simulink model "VCU_SW_1"  (R2023b)
settings: Solver=FixedStepDiscrete  StartTime=0.0  StopTime=inf  FixedStep=1e-2  RelTol=1e-3
PreLoadFcn:
  | RTWConfigurationCB('preloadfcn', bdroot);
InitFcn:
  | loadvar_ttc500
undefined symbols (not defined in the file): BrkPedalTypes, CabMovModeTypes, cFuseTempSensAcc_X, cFuseTempSensAcc_Y, cFuseTempSensVal_X, cFuseTempSensVal_Y, cTMSTempSensVal_X, cTMSTempSensVal_Y, cTransferCaseSpeedRatio, diag_state, DoorsPositionTypes, dP_filter_Y, DriverOccClassSystemTypes, ErrorValueTypes, fatal_error_callback, IO_ADC_NO_RANGE, LadderStatusTypes, pAnalogCabRotSensAcc, pAnalogCabRotSensMaxVolt, pAnalogCabRotSensMinVolt, pAnalogCabRotSensRange, pAnalogCabRotSensZeroVolt, pBrkActivePress, pCabTiltSensAcc, pCabTiltSensMaxCur, pCabTiltSensMinCur, pDistanceCorrection, pECANManual_BPNEnable, pECANManual_BPNEnabler_Flag, pFilterSensAccRes, pHDirMaxDiffFrq, pHDirSensHighLvl, pHDirSensLowLvl, pMainGearRatio, pMaxFilterSensRes, pMaxFirstPedalSensValue, pMaxFuseTempSensRes, pMaxPressLoss, pMaxPressSensCurrent, pMaxPressValue, pMaxPressValueHydMotAndPump, pMaxPressValueParkDrain, pMaxSecondPedalSensValue, pMaxTempSensVoltage, pMaxTempValue, pMaxTMSTempSensRes, pMinFilterSensRes, pMinFirstPedalSensValue, pMinFuseTempSensRes, pMinPressLoss, pMinPressSensCurrent, pMinPressValue, pMinSecondPedalSensValue, pMinTempSensVoltage, pMinTempValue, pMinTMSTempSensRes, pMotorRingTeethNum, pPedalSensAccuracyPct, pPedalSensAccuracyVolt, pPressLossTreshhold ... (+20)
libraries: TTlibrary x270, canmsglib x127, simulink x88
(part 11 of 19)

== system VCU_SW_1/logSignal/getListData/pageHighvoltageAppData/getListDataII8 ==
  getListDataII8 : TriggerPort  TriggerType=function-call  IsSimulinkFunction=on  FunctionName=getListDataII8  FunctionVisibility=scoped  VariantControl=(inherit)
  Constant : Constant  Value=uint8(6)
  Data Store Read1 : DataStoreRead  DataStoreName=sMinCellVoltage  IndexOptions=Index vector (dialog)  Indices=1  OutputSizes=1
  Data Store Read2 : DataStoreRead  DataStoreName=sMaxBatTemp  IndexOptions=Index vector (dialog)  Indices=1  OutputSizes=1
  Data Store Read3 : DataStoreRead  DataStoreName=sMinBatTemp  IndexOptions=Index vector (dialog)  Indices=1  OutputSizes=1
  Demux1 : Demux  Outputs=2
  Demux11 : Demux  Outputs=2
  Demux2 : Demux  Outputs=2
  Function Caller : FunctionCaller  FunctionPrototype=data = getListData.splitIntoTwoBytes(value)  InputArgumentSpecifications=<Enter example>  OutputArgumentSpecifications=<Enter example>
  Function Caller1 : FunctionCaller  FunctionPrototype=data = getListData.splitIntoTwoBytes(value)  InputArgumentSpecifications=<Enter example>  OutputArgumentSpecifications=<Enter example>
  Function Caller2 : FunctionCaller  FunctionPrototype=data = getListData.splitIntoTwoBytes(value)  InputArgumentSpecifications=<Enter example>  OutputArgumentSpecifications=<Enter example>
  Ground : Ground
  Mux : Mux  Inputs=7
  data : ArgOut  DisableCoverage=on  OutDataTypeStr=uint8  PortDimensions=[1,7]  ArgumentName=data
  len : ArgOut  Port=2  OutDataTypeStr=uint8  ArgumentName=len
  wires:
  Mux/1 -> data/1
  Constant/1 -> len/1
  Function Caller/1 -> Demux11/1
  Demux11/1 -> Mux/1
  Data Store Read1/1 -> Function Caller/1
  Demux11/2 -> Mux/2
  Demux1/2 -> Mux/4
  Data Store Read2/1 -> Function Caller1/1
  Demux1/1 -> Mux/3
  Function Caller1/1 -> Demux1/1
  Function Caller2/1 -> Demux2/1
  Demux2/2 -> Mux/6
  Demux2/1 -> Mux/5
  Ground/1 -> Mux/7
  Data Store Read3/1 -> Function Caller2/1

== system VCU_SW_1/logSignal/getListData/pageHighvoltageAppData/getListDataII9 ==
  getListDataII9 : TriggerPort  TriggerType=function-call  IsSimulinkFunction=on  FunctionName=getListDataII9  FunctionVisibility=scoped  VariantControl=(inherit)
  Constant : Constant  Value=uint8(6)
  Data Store Read1 : DataStoreRead  DataStoreName=sTotalVoltage  IndexOptions=Index vector (dialog)  Indices=1  OutputSizes=1
  Data Store Read2 : DataStoreRead  DataStoreName=sMaxCellVoltTemp  IndexOptions=Index vector (dialog)  Indices=1  OutputSizes=1
  Data Store Read3 : DataStoreRead  DataStoreName=sMinCellVoltTemp  IndexOptions=Index vector (dialog)  Indices=1  OutputSizes=1
  Data Store Read4 : DataStoreRead  DataStoreName=sSettingTargetWaterTemp  IndexOptions=Index vector (dialog)  Indices=1  OutputSizes=1
  Data Store Read5 : DataStoreRead  DataStoreName=sAverageBatTemp  IndexOptions=Index vector (dialog)  Indices=1  OutputSizes=1
  Demux11 : Demux  Outputs=2
  Function Caller : FunctionCaller  FunctionPrototype=data = getListData.splitIntoTwoBytes(value)  InputArgumentSpecifications=<Enter example>  OutputArgumentSpecifications=<Enter example>
  Ground : Ground
  Mux : Mux  Inputs=7
  data : ArgOut  DisableCoverage=on  OutDataTypeStr=uint8  PortDimensions=[1,7]  ArgumentName=data
  len : ArgOut  Port=2  OutDataTypeStr=uint8  ArgumentName=len
  wires:
  Data Store Read1/1 -> Function Caller/1
  Function Caller/1 -> Demux11/1
  Constant/1 -> len/1
  Mux/1 -> data/1
  Demux11/1 -> Mux/3
  Demux11/2 -> Mux/4
  Data Store Read3/1 -> Mux/2
  Data Store Read2/1 -> Mux/1
  Data Store Read4/1 -> Mux/5
  Data Store Read5/1 -> Mux/6
  Ground/1 -> Mux/7

== system VCU_SW_1/logSignal/getListData/pageOutputRawData/getListDataOI1 ==
  getListDataOI1 : TriggerPort  TriggerType=function-call  IsSimulinkFunction=on  FunctionName=getListDataOI1  FunctionVisibility=scoped  VariantControl=(inherit)
  Data Store Read2 : DataStoreRead  DataStoreName=sCoolSensSup  IndexOptions=Index vector (dialog)  Indices=1  OutputSizes=1
  Data Store Read3 : DataStoreRead  DataStoreName=sOnBrdChrgTermSttSup  IndexOptions=Index vector (dialog)  Indices=1  OutputSizes=1
  Data Store Read4 : DataStoreRead  DataStoreName=sHVILSup  IndexOptions=Index vector (dialog)  Indices=1  OutputSizes=1
  Data Store Read5 : DataStoreRead  DataStoreName=sOnBrdFastChrgSup  IndexOptions=Index vector (dialog)  Indices=1  OutputSizes=1
  Data Store Read6 : DataStoreRead  DataStoreName=sPressSensSup  IndexOptions=Index vector (dialog)  Indices=1  OutputSizes=1
  Data Store Read7 : DataStoreRead  DataStoreName=sGearboxSensSup  IndexOptions=Index vector (dialog)  Indices=1  OutputSizes=1
  Data Store Read8 : DataStoreRead  DataStoreName=sACDCChrgConvSwt  IndexOptions=Index vector (dialog)  Indices=1  OutputSizes=1
  Mux : Mux  Inputs=7
  data : ArgOut  DisableCoverage=on  OutDataTypeStr=uint8  PortDimensions=[1,7]  ArgumentName=data
  wires:
  Mux/1 -> data/1
  Data Store Read2/1 -> Mux/7
  Data Store Read3/1 -> Mux/6
  Data Store Read8/1 -> Mux/1
  Data Store Read4/1 -> Mux/5
  Data Store Read7/1 -> Mux/2
  Data Store Read5/1 -> Mux/4
  Data Store Read6/1 -> Mux/3

== system VCU_SW_1/logSignal/getListData/pageOutputRawData/getListDataOI2 ==
  getListDataOI2 : TriggerPort  TriggerType=function-call  IsSimulinkFunction=on  FunctionName=getListDataOI2  FunctionVisibility=scoped  VariantControl=(inherit)
  Data Store Read : DataStoreRead  DataStoreName=sCapsSup  IndexOptions=Index vector (dialog)  Indices=1  OutputSizes=1
  Data Store Read1 : DataStoreRead  DataStoreName=sPumpFlowSetPnt  IndexOptions=Index vector (dialog)  Indices=1  OutputSizes=1
  Data Store Read12 : DataStoreRead  DataStoreName=sTMSComprSetPnt  IndexOptions=Index vector (dialog)  Indices=1  OutputSizes=1
  Data Store Read13 : DataStoreRead  DataStoreName=sCircPumpSetPnt  IndexOptions=Index vector (dialog)  Indices=1  OutputSizes=1
  Demux : Demux  Outputs=2
  Demux1 : Demux  Outputs=2
  Demux2 : Demux  Outputs=2
  Function Caller3 : FunctionCaller  FunctionPrototype=data = getListData.splitIntoTwoBytes(value)  InputArgumentSpecifications=<Enter example>  OutputArgumentSpecifications=<Enter example>
  Function Caller4 : FunctionCaller  FunctionPrototype=data = getListData.splitIntoTwoBytes(value)  InputArgumentSpecifications=<Enter example>  OutputArgumentSpecifications=<Enter example>
  Function Caller5 : FunctionCaller  FunctionPrototype=data = getListData.splitIntoTwoBytes(value)  InputArgumentSpecifications=<Enter example>  OutputArgumentSpecifications=<Enter example>
  Mux1 : Mux  Inputs=7
  data : ArgOut  DisableCoverage=on  OutDataTypeStr=uint8  PortDimensions=[1,7]  ArgumentName=data
  wires:
  Mux1/1 -> data/1
  Data Store Read12/1 -> Function Caller4/1
  Demux1/1 -> Mux1/3
  Demux/2 -> Mux1/2
  Demux2/1 -> Mux1/5
  Demux/1 -> Mux1/1
  Data Store Read13/1 -> Function Caller5/1
  Demux2/2 -> Mux1/6
  Function Caller3/1 -> Demux/1
  Data Store Read1/1 -> Function Caller3/1
  Data Store Read/1 -> Mux1/7
  Demux1/2 -> Mux1/4
  Function Caller4/1 -> Demux1/1
  Function Caller5/1 -> Demux2/1

== system VCU_SW_1/logSignal/getListData/pageOutputRawData/getListDataOI3 ==
  getListDataOI3 : TriggerPort  TriggerType=function-call  IsSimulinkFunction=on  FunctionName=getListDataOI3  FunctionVisibility=scoped  VariantControl=(inherit)
  Data Store Read10 : DataStoreRead  DataStoreName=sSecondGearVlvSetPnt  IndexOptions=Index vector (dialog)  Indices=1  OutputSizes=1
  Data Store Read11 : DataStoreRead  DataStoreName=sRemBrkVlvSetPnt  IndexOptions=Index vector (dialog)  Indices=1  OutputSizes=1
  Data Store Read9 : DataStoreRead  DataStoreName=sFirstGearVlvSetPnt  IndexOptions=Index vector (dialog)  Indices=1  OutputSizes=1
  Demux3 : Demux  Outputs=2
  Demux4 : Demux  Outputs=2
  Demux5 : Demux  Outputs=2
  Function Caller : FunctionCaller  FunctionPrototype=data = getListData.splitIntoTwoBytes(value)  InputArgumentSpecifications=<Enter example>  OutputArgumentSpecifications=<Enter example>
  Function Caller1 : FunctionCaller  FunctionPrototype=data = getListData.splitIntoTwoBytes(value)  InputArgumentSpecifications=<Enter example>  OutputArgumentSpecifications=<Enter example>
  Function Caller2 : FunctionCaller  FunctionPrototype=data = getListData.splitIntoTwoBytes(value)  InputArgumentSpecifications=<Enter example>  OutputArgumentSpecifications=<Enter example>
  Ground : Ground
  Mux2 : Mux  Inputs=7
  data : ArgOut  DisableCoverage=on  OutDataTypeStr=uint8  PortDimensions=[1,7]  ArgumentName=data
  wires:
  Function Caller1/1 -> Demux4/1
  Function Caller2/1 -> Demux5/1
  Demux4/2 -> Mux2/4
  Demux3/2 -> Mux2/2
  Demux5/1 -> Mux2/5
  Demux3/1 -> Mux2/1
  Demux4/1 -> Mux2/3
  Data Store Read9/1 -> Function Caller/1
  Data Store Read10/1 -> Function Caller1/1
  Ground/1 -> Mux2/7
  Function Caller/1 -> Demux3/1
  Demux5/2 -> Mux2/6
  Data Store Read11/1 -> Function Caller2/1
  Mux2/1 -> data/1

== system VCU_SW_1/logSignal/getListData/pageRawInput/getListDataII1 ==
  getListDataII1 : TriggerPort  TriggerType=function-call  IsSimulinkFunction=on  FunctionName=getListDataII1  FunctionVisibility=scoped  VariantControl=(inherit)
  Constant : Constant  Value=uint8(7)
  Data Store Read1 : DataStoreRead  DataStoreName=sHVILSup  IndexOptions=Index vector (dialog)  Indices=1  OutputSizes=1
  Data Store Read2 : DataStoreRead  DataStoreName=sPrechargeCtrlStt  IndexOptions=Index vector (dialog)  Indices=1  OutputSizes=1
  Data Store Read3 : DataStoreRead  DataStoreName=sDCDCEmergGND  IndexOptions=Index vector (dialog)  Indices=1  OutputSizes=1
  Data Store Read4 : DataStoreRead  DataStoreName=sACChrgSupTermStt  IndexOptions=Index vector (dialog)  Indices=1  OutputSizes=1
  Data Store Read5 : DataStoreRead  DataStoreName=sACChrgGndTermStt  IndexOptions=Index vector (dialog)  Indices=1  OutputSizes=1
  Data Store Read6 : DataStoreRead  DataStoreName=sDCChrgSupTermStt  IndexOptions=Index vector (dialog)  Indices=1  OutputSizes=1
  Data Store Read7 : DataStoreRead  DataStoreName=sDCChrgGndTermStt  IndexOptions=Index vector (dialog)  Indices=1  OutputSizes=1
  Mux : Mux  Inputs=7
  data : ArgOut  DisableCoverage=on  OutDataTypeStr=uint8  PortDimensions=[1,7]  ArgumentName=data
  len : ArgOut  Port=2  OutDataTypeStr=uint8  ArgumentName=len
  wires:
  Data Store Read5/1 -> Mux/4
  Data Store Read2/1 -> Mux/7
  Data Store Read3/1 -> Mux/5
  Data Store Read7/1 -> Mux/3
  Data Store Read4/1 -> Mux/1
  Data Store Read6/1 -> Mux/2
  Data Store Read1/1 -> Mux/6
  Mux/1 -> data/1
  Constant/1 -> len/1

== system VCU_SW_1/logSignal/getListData/pageRawInput/getListDataII2 ==
  getListDataII2 : TriggerPort  TriggerType=function-call  IsSimulinkFunction=on  FunctionName=getListDataII2  FunctionVisibility=scoped  VariantControl=(inherit)
  Constant : Constant  Value=uint8(7)
  Data Store Read : DataStoreRead  DataStoreName=sGlobalSupTermStt  IndexOptions=Index vector (dialog)  Indices=1  OutputSizes=1
  Data Store Read10 : DataStoreRead  DataStoreName=sFrontCargoWeight  IndexOptions=Index vector (dialog)  Indices=1  OutputSizes=1
  Data Store Read11 : DataStoreRead  DataStoreName=sRearCargoWeight  IndexOptions=Index vector (dialog)  Indices=1  OutputSizes=1
  Data Store Read14 : DataStoreRead  DataStoreName=sGearboxOilState  IndexOptions=Index vector (dialog)  Indices=1  OutputSizes=1
  Demux : Demux  Outputs=2
  Demux1 : Demux  Outputs=2
  Demux2 : Demux  Outputs=2
  Function Caller : FunctionCaller  FunctionPrototype=data = getListData.splitIntoTwoBytes(value)  InputArgumentSpecifications=<Enter example>  OutputArgumentSpecifications=<Enter example>
  Function Caller13 : FunctionCaller  FunctionPrototype=data = getListData.splitIntoTwoBytes(value)  InputArgumentSpecifications=<Enter example>  OutputArgumentSpecifications=<Enter example>
  Function Caller14 : FunctionCaller  FunctionPrototype=data = getListData.splitIntoTwoBytes(value)  InputArgumentSpecifications=<Enter example>  OutputArgumentSpecifications=<Enter example>
  Mux1 : Mux  Inputs=7
  data : ArgOut  DisableCoverage=on  OutDataTypeStr=uint8  PortDimensions=[1,7]  ArgumentName=data
  len : ArgOut  Port=2  OutDataTypeStr=uint8  ArgumentName=len
  wires:
  Data Store Read/1 -> Mux1/7
  Data Store Read14/1 -> Function Caller/1
  Demux2/2 -> Mux1/6
  Demux2/1 -> Mux1/5
  Demux/2 -> Mux1/2
  Data Store Read10/1 -> Function Caller13/1
  Demux/1 -> Mux1/1
  Function Caller/1 -> Demux/1
  Function Caller13/1 -> Demux1/1
  Demux1/1 -> Mux1/3
  Demux1/2 -> Mux1/4
  Function Caller14/1 -> Demux2/1
  Data Store Read11/1 -> Function Caller14/1
  Mux1/1 -> data/1
  Constant/1 -> len/1

== system VCU_SW_1/logSignal/getListData/pageRawInput/getListDataII3 ==
  getListDataII3 : TriggerPort  TriggerType=function-call  IsSimulinkFunction=on  FunctionName=getListDataII3  FunctionVisibility=scoped  VariantControl=(inherit)
  Constant : Constant  Value=uint8(6)
  Data Store Read12 : DataStoreRead  DataStoreName=sTMSTempInput  IndexOptions=Index vector (dialog)  Indices=1  OutputSizes=1
  Data Store Read17 : DataStoreRead  DataStoreName=sPumpFlowCur  IndexOptions=Index vector (dialog)  Indices=1  OutputSizes=1
  Demux3 : Demux
  Demux4 : Demux  Outputs=2
  Function Caller1 : FunctionCaller  FunctionPrototype=data = getListData.splitIntoFourBytes(value)  InputArgumentSpecifications=<Enter example>  OutputArgumentSpecifications=<Enter example>
  Function Caller2 : FunctionCaller  FunctionPrototype=data = getListData.splitIntoTwoBytes(value)  InputArgumentSpecifications=<Enter example>  OutputArgumentSpecifications=<Enter example>
  Ground : Ground
  Mux2 : Mux  Inputs=7
  data : ArgOut  DisableCoverage=on  OutDataTypeStr=uint8  PortDimensions=[1,7]  ArgumentName=data
  len : ArgOut  Port=2  OutDataTypeStr=uint8  ArgumentName=len
  wires:
  Demux4/2 -> Mux2/6
  Ground/1 -> Mux2/7
  Demux3/4 -> Mux2/4
  Demux3/2 -> Mux2/2
  Function Caller2/1 -> Demux4/1
  Data Store Read17/1 -> Function Caller2/1
  Demux3/1 -> Mux2/1
  Demux4/1 -> Mux2/5
  Function Caller1/1 -> Demux3/1
  Data Store Read12/1 -> Function Caller1/1
  Demux3/3 -> Mux2/3
  Mux2/1 -> data/1
  Constant/1 -> len/1

== system VCU_SW_1/logSignal/getListData/pageRawInput/getListDataII4 ==
  getListDataII4 : TriggerPort  TriggerType=function-call  IsSimulinkFunction=on  FunctionName=getListDataII4  FunctionVisibility=scoped  VariantControl=(inherit)
  Constant : Constant  Value=uint8(6)
  Data Store Read13 : DataStoreRead  DataStoreName=sTMSTempOutput  IndexOptions=Index vector (dialog)  Indices=1  OutputSizes=1
  Data Store Read18 : DataStoreRead  DataStoreName=sFirstGearVlvCur  IndexOptions=Index vector (dialog)  Indices=1  OutputSizes=1
  Demux5 : Demux
  Demux6 : Demux  Outputs=2
  Function Caller3 : FunctionCaller  FunctionPrototype=data = getListData.splitIntoTwoBytes(value)  InputArgumentSpecifications=<Enter example>  OutputArgumentSpecifications=<Enter example>
  Function Caller8 : FunctionCaller  FunctionPrototype=data = getListData.splitIntoFourBytes(value)  InputArgumentSpecifications=<Enter example>  OutputArgumentSpecifications=<Enter example>
  Ground1 : Ground
  Mux3 : Mux  Inputs=7
  data : ArgOut  DisableCoverage=on  OutDataTypeStr=uint8  PortDimensions=[1,7]  ArgumentName=data
  len : ArgOut  Port=2  OutDataTypeStr=uint8  ArgumentName=len
  wires:
  Function Caller8/1 -> Demux5/1
  Function Caller3/1 -> Demux6/1
  Data Store Read13/1 -> Function Caller8/1
  Demux6/2 -> Mux3/6
  Demux6/1 -> Mux3/5
  Data Store Read18/1 -> Function Caller3/1
  Demux5/2 -> Mux3/2
  Demux5/3 -> Mux3/3
  Demux5/4 -> Mux3/4
  Demux5/1 -> Mux3/1
  Ground1/1 -> Mux3/7
  Mux3/1 -> data/1
  Constant/1 -> len/1

== system VCU_SW_1/logSignal/getListData/pageRawInput/getListDataII5 ==
  getListDataII5 : TriggerPort  TriggerType=function-call  IsSimulinkFunction=on  FunctionName=getListDataII5  FunctionVisibility=scoped  VariantControl=(inherit)
  Constant : Constant  Value=uint8(6)
  Data Store Read19 : DataStoreRead  DataStoreName=sSecondGearVlvCur  IndexOptions=Index vector (dialog)  Indices=1  OutputSizes=1
  Data Store Read8 : DataStoreRead  DataStoreName=sFuseBoxTempSens1  IndexOptions=Index vector (dialog)  Indices=1  OutputSizes=1
  Demux7 : Demux
  Demux8 : Demux  Outputs=2
  Function Caller4 : FunctionCaller  FunctionPrototype=data = getListData.splitIntoTwoBytes(value)  InputArgumentSpecifications=<Enter example>  OutputArgumentSpecifications=<Enter example>
  Function Caller9 : FunctionCaller  FunctionPrototype=data = getListData.splitIntoFourBytes(value)  InputArgumentSpecifications=<Enter example>  OutputArgumentSpecifications=<Enter example>
  Ground2 : Ground
  Mux4 : Mux  Inputs=7
  data : ArgOut  DisableCoverage=on  OutDataTypeStr=uint8  PortDimensions=[1,7]  ArgumentName=data
  len : ArgOut  Port=2  OutDataTypeStr=uint8  ArgumentName=len
  wires:
  Function Caller9/1 -> Demux7/1
  Data Store Read19/1 -> Function Caller4/1
  Ground2/1 -> Mux4/7
  Demux8/2 -> Mux4/6
  Demux7/4 -> Mux4/4
  Demux7/1 -> Mux4/1
  Demux7/3 -> Mux4/3
  Function Caller4/1 -> Demux8/1
  Demux7/2 -> Mux4/2
  Demux8/1 -> Mux4/5
  Data Store Read8/1 -> Function Caller9/1
  Mux4/1 -> data/1
  Constant/1 -> len/1

== system VCU_SW_1/logSignal/getListData/pageRawInput/getListDataII6 ==
  getListDataII6 : TriggerPort  TriggerType=function-call  IsSimulinkFunction=on  FunctionName=getListDataII6  FunctionVisibility=scoped  VariantControl=(inherit)
  Constant : Constant  Value=uint8(6)
  Data Store Read20 : DataStoreRead  DataStoreName=sRemBrkVlvCur  IndexOptions=Index vector (dialog)  Indices=1  OutputSizes=1
  Data Store Read9 : DataStoreRead  DataStoreName=sFuseBoxTempSens2  IndexOptions=Index vector (dialog)  Indices=1  OutputSizes=1
  Demux10 : Demux  Outputs=2
  Demux9 : Demux
  Function Caller10 : FunctionCaller  FunctionPrototype=data = getListData.splitIntoFourBytes(value)  InputArgumentSpecifications=<Enter example>  OutputArgumentSpecifications=<Enter example>
  Function Caller5 : FunctionCaller  FunctionPrototype=data = getListData.splitIntoTwoBytes(value)  InputArgumentSpecifications=<Enter example>  OutputArgumentSpecifications=<Enter example>
  Ground3 : Ground
  Mux5 : Mux  Inputs=7
  data : ArgOut  DisableCoverage=on  OutDataTypeStr=uint8  PortDimensions=[1,7]  ArgumentName=data
  len : ArgOut  Port=2  OutDataTypeStr=uint8  ArgumentName=len
  wires:
  Function Caller10/1 -> Demux9/1
  Data Store Read20/1 -> Function Caller5/1
  Demux9/2 -> Mux5/2
  Demux9/3 -> Mux5/3
  Demux9/1 -> Mux5/1
  Demux10/2 -> Mux5/6
  Ground3/1 -> Mux5/7
  Function Caller5/1 -> Demux10/1
  Demux10/1 -> Mux5/5
  Data Store Read9/1 -> Function Caller10/1
  Demux9/4 -> Mux5/4
  Mux5/1 -> data/1
  Constant/1 -> len/1

== system VCU_SW_1/logSignal/getListData/pageRawInput/getListDataII7 ==
  getListDataII7 : TriggerPort  TriggerType=function-call  IsSimulinkFunction=on  FunctionName=getListDataII7  FunctionVisibility=scoped  VariantControl=(inherit)
  Constant : Constant  Value=uint8(6)
  Data Store Read15 : DataStoreRead  DataStoreName=sOutShaftFreq  IndexOptions=Index vector (dialog)  Indices=1  OutputSizes=1
  Data Store Read21 : DataStoreRead  DataStoreName=sTMSComprCur  IndexOptions=Index vector (dialog)  Indices=1  OutputSizes=1
  Demux11 : Demux  Outputs=2
  Demux12 : Demux
  Function Caller11 : FunctionCaller  FunctionPrototype=data = getListData.splitIntoFourBytes(value)  InputArgumentSpecifications=<Enter example>  OutputArgumentSpecifications=<Enter example>
  Function Caller7 : FunctionCaller  FunctionPrototype=data = getListData.splitIntoTwoBytes(value)  InputArgumentSpecifications=<Enter example>  OutputArgumentSpecifications=<Enter example>
  Ground4 : Ground
  Mux6 : Mux  Inputs=7
  data : ArgOut  DisableCoverage=on  OutDataTypeStr=uint8  PortDimensions=[1,7]  ArgumentName=data
  len : ArgOut  Port=2  OutDataTypeStr=uint8  ArgumentName=len
  wires:
  Function Caller7/1 -> Demux11/1
  Function Caller11/1 -> Demux12/1
  Demux11/2 -> Mux6/6
  Ground4/1 -> Mux6/7
  Demux12/4 -> Mux6/4
  Demux11/1 -> Mux6/5
  Demux12/2 -> Mux6/2
  Data Store Read21/1 -> Function Caller7/1
  Data Store Read15/1 -> Function Caller11/1
  Demux12/1 -> Mux6/1
  Demux12/3 -> Mux6/3
  Mux6/1 -> data/1
  Constant/1 -> len/1

== system VCU_SW_1/logSignal/getListData/pageRawInput/getListDataII8 ==
  getListDataII8 : TriggerPort  TriggerType=function-call  IsSimulinkFunction=on  FunctionName=getListDataII8  FunctionVisibility=scoped  VariantControl=(inherit)
  Constant : Constant  Value=uint8(6)
  Data Store Read16 : DataStoreRead  DataStoreName=sRingShaftFreq  IndexOptions=Index vector (dialog)  Indices=1  OutputSizes=1
  Data Store Read22 : DataStoreRead  DataStoreName=sCircPumpCur  IndexOptions=Index vector (dialog)  Indices=1  OutputSizes=1
  Demux13 : Demux  Outputs=2
  Demux14 : Demux
  Function Caller12 : FunctionCaller  FunctionPrototype=data = getListData.splitIntoFourBytes(value)  InputArgumentSpecifications=<Enter example>  OutputArgumentSpecifications=<Enter example>
  Function Caller6 : FunctionCaller  FunctionPrototype=data = getListData.splitIntoTwoBytes(value)  InputArgumentSpecifications=<Enter example>  OutputArgumentSpecifications=<Enter example>
  Ground5 : Ground
  Mux7 : Mux  Inputs=7
  data : ArgOut  DisableCoverage=on  OutDataTypeStr=uint8  PortDimensions=[1,7]  ArgumentName=data
  len : ArgOut  Port=2  OutDataTypeStr=uint8  ArgumentName=len
  wires:
  Function Caller6/1 -> Demux13/1
  Demux14/3 -> Mux7/3
  Data Store Read16/1 -> Function Caller12/1
  Demux13/1 -> Mux7/5
  Function Caller12/1 -> Demux14/1
  Data Store Read22/1 -> Function Caller6/1
  Demux14/2 -> Mux7/2
  Demux14/4 -> Mux7/4
  Demux13/2 -> Mux7/6
  Ground5/1 -> Mux7/7
  Demux14/1 -> Mux7/1
  Mux7/1 -> data/1
  Constant/1 -> len/1

== system VCU_SW_1/InputLayer/InputInterfaces/AnalogInput/AIProc1000msec/Filter ==
  note: Просто сделать статус загрязнено или не загрязнено
  1-D Lookup Table : Lookup_n-D  Commented=on  NumberOfTableDimensions=1  BreakpointsForDimension1=res_filter_X  Table=dP_filter_Y  InternalRulePriority=Speed  RndMeth=Simplest
  Constant1 : Constant  Value=pMaxPressLoss
  Constant12 : Constant  Value=pFilterSensAccRes
  Constant2 : Constant  Value=pMinPressLoss
  Constant3 : Constant  Value=pPressLossTreshhold
  Constant8 : Constant  Value=pMaxFilterSensRes
  Constant9 : Constant  Value=pMinFilterSensRes
  Data Store Read11 : DataStoreRead  DataStoreName=InputInterfaceData  DataStoreElements=InputInterfaceData.AI.filterClogSens  IndexOptions=Index vector (dialog)  Indices=1  OutputSizes=1
  Data Store Write14 : DataStoreWrite  DataStoreName=InputFunctionsData  DataStoreElements=InputFunctionsData.filterPollutionState  IndexOptions=Index vector (dialog)  Indices=1  OutputSizes=1
  MATLAB Function1 : MATLAB Function  TreatAsAtomicUnit=on
  wires:
  Constant8/1 -> MATLAB Function1/1(maxRes)
  Constant9/1 -> MATLAB Function1/2(minRes)
  Constant12/1 -> MATLAB Function1/4(accuracyValue)
  Data Store Read11/1 -> MATLAB Function1/3(sensorValue)
  Constant1/1 -> MATLAB Function1/5(maxPress)
  Constant2/1 -> MATLAB Function1/6(minPress)
  MATLAB Function1/1(filterState) -> Data Store Write14/1
  Constant3/1 -> MATLAB Function1/7(Treshold)

== system VCU_SW_1/InputLayer/InputInterfaces/AnalogInput/AIProc1000msec/TemperatureValues ==
  Constant1 : Constant  Value=pMinTempValue
  Constant16 : Constant  Value=pMinTempValue
  Constant2 : Constant  Value=pMaxTempValue
  Constant28 : Constant  Value=pMaxTempValue
  Data Store Read1 : DataStoreRead  DataStoreName=InputInterfaceData  DataStoreElements=InputInterfaceData.AI.transPumpTempSens  IndexOptions=Index vector (dialog)  Indices=1  OutputSizes=1
  Data Store Read13 : DataStoreRead  DataStoreName=InputInterfaceData  DataStoreElements=InputInterfaceData.AI.hydMotTempSens  IndexOptions=Index vector (dialog)  Indices=1  OutputSizes=1
  Data Store Write1 : DataStoreWrite  DataStoreName=InputFunctionsData  DataStoreElements=InputFunctionsData.transPumpTemperature  IndexOptions=Index vector (dialog)  Indices=1  OutputSizes=1
  Data Store Write14 : DataStoreWrite  DataStoreName=InputFunctionsData  DataStoreElements=InputFunctionsData.hydMotTemperature  IndexOptions=Index vector (dialog)  Indices=1  OutputSizes=1
  Data Store Write2 : DataStoreWrite  DataStoreName=UDSStruct  DataStoreElements=UDSStruct.transPumpTempSens  IndexOptions=Index vector (dialog)  Indices=1  OutputSizes=1
  Data Store Write4 : DataStoreWrite  DataStoreName=UDSStruct  DataStoreElements=UDSStruct.hydMotTempSens  IndexOptions=Index vector (dialog)  Indices=1  OutputSizes=1
  Function Caller : FunctionCaller  FunctionPrototype=tempValue = TemperatureValues.calcCurPressSens(sensValue,tempMax,tempMin)  InputArgumentSpecifications=<Enter example>  OutputArgumentSpecifications=<Enter example>
  Function Caller1 : FunctionCaller  FunctionPrototype=tempValue = TemperatureValues.calcCurPressSens(sensValue,tempMax,tempMin)  InputArgumentSpecifications=<Enter example>  OutputArgumentSpecifications=<Enter example>
  calcCurPressSensVal : Subsystem  TreatAsAtomicUnit=on
  calcFuseTemp : Subsystem  Commented=on  TreatAsAtomicUnit=on
  calcTMSTemp : Subsystem  Commented=on  TreatAsAtomicUnit=on
  wires:
  Function Caller1/1 -> Data Store Write1/1, Data Store Write2/1
  Function Caller/1 -> Data Store Write14/1, Data Store Write4/1
  Constant16/1 -> Function Caller/3
  Constant28/1 -> Function Caller/2
  Data Store Read13/1 -> Function Caller/1
  Data Store Read1/1 -> Function Caller1/1
  Constant2/1 -> Function Caller1/2
  Constant1/1 -> Function Caller1/3

== system VCU_SW_1/InputLayer/InputInterfaces/AnalogInput/AIProc100msec/GenWorkSig ==
  Data Store Read : DataStoreRead  DataStoreName=InputInterfaceData  DataStoreElements=InputInterfaceData.AI.upperGenWorkSig  IndexOptions=Index vector (dialog)  Indices=1  OutputSizes=1
  Data Store Read1 : DataStoreRead  DataStoreName=InputInterfaceData  DataStoreElements=InputInterfaceData.AI.lowerGenWorkSig  IndexOptions=Index vector (dialog)  Indices=1  OutputSizes=1
  Data Store Write : DataStoreWrite  DataStoreName=InputFunctionsData  DataStoreElements=InputFunctionsData.upperGenWorkSignal  IndexOptions=Index vector (dialog)  Indices=1  OutputSizes=1
  Data Store Write1 : DataStoreWrite  DataStoreName=InputFunctionsData  DataStoreElements=InputFunctionsData.lowerGenWorkSignal  IndexOptions=Index vector (dialog)  Indices=1  OutputSizes=1
  Function Caller : FunctionCaller  FunctionPrototype=finalState = voltageAIConv(Volt)  InputArgumentSpecifications=<Enter example>  OutputArgumentSpecifications=<Enter example>
  Function Caller1 : FunctionCaller  FunctionPrototype=finalState = voltageAIConv(Volt)  InputArgumentSpecifications=<Enter example>  OutputArgumentSpecifications=<Enter example>
  wires:
  Data Store Read/1 -> Function Caller/1
  Data Store Read1/1 -> Function Caller1/1
  Function Caller/1 -> Data Store Write/1
  Function Caller1/1 -> Data Store Write1/1

== system VCU_SW_1/InputLayer/InputInterfaces/AnalogInput/AIProc100msec/PressureValues ==
  Constant10 : Constant  Value=pMaxPressValue
  Constant11 : Constant  Value=pMaxPressValue
  Constant13 : Constant  Value=pMinPressValue
  Constant14 : Constant  Value=pMinPressValue
  Constant15 : Constant  Value=pMinPressValue
  Constant24 : Constant  Value=pMaxPressValueParkDrain
  Data Store Read10 : DataStoreRead  DataStoreName=InputInterfaceData  DataStoreElements=InputInterfaceData.AI.brkSupplyFrontPressSens  IndexOptions=Index vector (dialog)  Indices=1  OutputSizes=1
  Data Store Read11 : DataStoreRead  DataStoreName=InputInterfaceData  DataStoreElements=InputInterfaceData.AI.brkSupplyParkPressSens  IndexOptions=Index vector (dialog)  Indices=1  OutputSizes=1
  Data Store Read9 : DataStoreRead  DataStoreName=InputInterfaceData  DataStoreElements=InputInterfaceData.AI.brkSupplyRearPressSens  IndexOptions=Index vector (dialog)  Indices=1  OutputSizes=1
  Data Store Write10 : DataStoreWrite  DataStoreName=InputFunctionsData  DataStoreElements=InputFunctionsData.supplyRearBrakePressure  IndexOptions=Index vector (dialog)  Indices=1  OutputSizes=1
  Data Store Write11 : DataStoreWrite  DataStoreName=InputFunctionsData  DataStoreElements=InputFunctionsData.supplyFrontBrakePressure  IndexOptions=Index vector (dialog)  Indices=1  OutputSizes=1
  Data Store Write12 : DataStoreWrite  DataStoreName=InputFunctionsData  DataStoreElements=InputFunctionsData.supplyParkBrakePressure  IndexOptions=Index vector (dialog)  Indices=1  OutputSizes=1
  Data Store Write3 : DataStoreWrite  DataStoreName=UDSStruct  DataStoreElements=UDSStruct.brkSupplyRearPressSens  IndexOptions=Index vector (dialog)  Indices=1  OutputSizes=1
  Data Store Write4 : DataStoreWrite  DataStoreName=UDSStruct  DataStoreElements=UDSStruct.brkSupplyFrontPressSens  IndexOptions=Index vector (dialog)  Indices=1  OutputSizes=1
  Data Store Write5 : DataStoreWrite  DataStoreName=UDSStruct  DataStoreElements=UDSStruct.brkSupplyParkPressSens  IndexOptions=Index vector (dialog)  Indices=1  OutputSizes=1
  Data Type Conversion : DataTypeConversion  OutDataTypeStr=uint16  SaturateOnIntegerOverflow=off  RndMeth=Floor
  Data Type Conversion1 : DataTypeConversion  OutDataTypeStr=uint16  SaturateOnIntegerOverflow=off  RndMeth=Floor
  Data Type Conversion2 : DataTypeConversion  OutDataTypeStr=uint16  SaturateOnIntegerOverflow=off  RndMeth=Floor
  Function Caller : FunctionCaller  FunctionPrototype=pressValue = PressureValues.calcCurPressSens(sensValue,pressMax,pressMin)  InputArgumentSpecifications=<Enter example>  OutputArgumentSpecifications=<Enter example>
  Function Caller11 : FunctionCaller  FunctionPrototype=pressValue = PressureValues.calcCurPressSens(sensValue,pressMax,pressMin)  InputArgumentSpecifications=<Enter example>  OutputArgumentSpecifications=<Enter example>
  Function Caller8 : FunctionCaller  FunctionPrototype=pressValue = PressureValues.calcCurPressSens(sensValue,pressMax,pressMin)  InputArgumentSpecifications=<Enter example>  OutputArgumentSpecifications=<Enter example>
  Gain : Gain  Gain=1/1000  OutDataTypeStr=Inherit: Same as input
  Gain1 : Gain  Gain=1/1000  OutDataTypeStr=Inherit: Same as input
  Gain2 : Gain  Gain=1/1000  OutDataTypeStr=Inherit: Same as input
  calcCurPressSensVal : Subsystem  TreatAsAtomicUnit=on
  wires:
  Function Caller11/1 -> Gain2/1, Data Store Write12/1
  Function Caller8/1 -> Gain1/1, Data Store Write11/1
  Function Caller/1 -> Data Store Write10/1, Gain/1
  Constant15/1 -> Function Caller11/3
  Data Store Read11/1 -> Function Caller11/1
  Constant24/1 -> Function Caller11/2
  Constant14/1 -> Function Caller8/3
  Data Store Read10/1 -> Function Caller8/1
  Constant11/1 -> Function Caller8/2
  Data Store Read9/1 -> Function Caller/1
  Constant10/1 -> Function Caller/2
  Constant13/1 -> Function Caller/3
  Gain/1 -> Data Type Conversion/1
  Data Type Conversion/1 -> Data Store Write3/1
  Gain1/1 -> Data Type Conversion1/1
  Data Type Conversion1/1 -> Data Store Write4/1
  Gain2/1 -> Data Type Conversion2/1
  Data Type Conversion2/1 -> Data Store Write5/1

== system VCU_SW_1/InputLayer/InputInterfaces/AnalogInput/AIProc10msec/CabMovValues ==
  note: две одинаковых функции в разных подсистемах, в чем проблема вытянуть их наверх и сделать одну?
  note: Если в датчик выдает пилу, то он может выкинуть ошибку в момент скачка, если он будет неодновременным в каналах
  function : TriggerPort  TriggerType=function-call  VariantControl=Variant
  Constant2 : Constant  Value=pResetCabTiltSensErr
  Constant3 : Constant  Value=pResetAnalogCabRotSensErr
  Constant4 : Constant  Value=pResetFrameTiltSensErr
  Data Store Read : DataStoreRead  DataStoreName=InputInterfaceData  DataStoreElements=InputInterfaceData.AI.cabTiltLeftTransSens  IndexOptions=Index vector (dialog)  Indices=1  OutputSizes=1
  Data Store Read1 : DataStoreRead  DataStoreName=InputInterfaceData  DataStoreElements=InputInterfaceData.AI.longitudinalTransPlatfAngleSens  IndexOptions=Index vector (dialog)  Indices=1  OutputSizes=1
  Data Store Read2 : DataStoreRead  DataStoreName=InputInterfaceData  DataStoreElements=InputInterfaceData.AI.transverseTransPlatfAngleSens  IndexOptions=Index vector (dialog)  Indices=1  OutputSizes=1
  Data Store Read3 : DataStoreRead  DataStoreName=InputInterfaceData  DataStoreElements=InputInterfaceData.AI.cabTiltLeftLongSens  IndexOptions=Index vector (dialog)  Indices=1  OutputSizes=1
  Simulink Function : Subsystem  TreatAsAtomicUnit=on
  Simulink Function1 : Subsystem  TreatAsAtomicUnit=on
  cabRotAnalogSensProc fcn : MATLAB Function  TreatAsAtomicUnit=on
  cabTiltSensProc fcn : MATLAB Function  TreatAsAtomicUnit=on
  frameTiltSensProc fcn : MATLAB Function  TreatAsAtomicUnit=on
  getAnalogCabRotSensData : Subsystem  TreatAsAtomicUnit=on
  getCabTiltSensData : Subsystem  TreatAsAtomicUnit=on
  setAnalogCabRotSensData : Subsystem  TreatAsAtomicUnit=on
  setAnalogSensErr : Subsystem  TreatAsAtomicUnit=on
  setCabTiltSensData : Subsystem  TreatAsAtomicUnit=on
  setCabTiltSensErr : Subsystem  TreatAsAtomicUnit=on
  setFrameTiltSensData : Subsystem  TreatAsAtomicUnit=on
  setFrameTiltSensErr : Subsystem  TreatAsAtomicUnit=on
  wires:
  Constant2/1 -> cabTiltSensProc fcn/1(pResetCabTiltSensErr)
  Constant4/1 -> frameTiltSensProc fcn/1(pResetFrameTiltSensErr)
  Constant3/1 -> cabRotAnalogSensProc fcn/1(pResetAnalogCabRotSensErr)
  Data Store Read3/1 -> cabTiltSensProc fcn/2(pitchSens)
  Data Store Read/1 -> cabTiltSensProc fcn/3(rollSens)
  Data Store Read1/1 -> frameTiltSensProc fcn/2(pitchSens)
  Data Store Read2/1 -> frameTiltSensProc fcn/3(rollSens)

== system VCU_SW_1/InputLayer/InputInterfaces/AnalogInput/AIProc10msec/PedalValues ==
  note: педалька на мануал (кан - ограничение, плавное наращивание, мб шаг наращивания)
  note: Acceleration Pedal
  Constant : Constant  Value=pMaxSecondPedalSensValue
  Constant1 : Constant  Value=pMinSecondPedalSensValue
  Constant2 : Constant  Value=pMaxFirstPedalSensValue
  Constant3 : Constant  Value=pMinFirstPedalSensValue
  Data Store Read : DataStoreRead  DataStoreName=InputInterfaceData  DataStoreElements=InputInterfaceData.AI.accPedSens1  IndexOptions=Index vector (dialog)  Indices=1  OutputSizes=1
  Data Store Read1 : DataStoreRead  DataStoreName=InputInterfaceData  DataStoreElements=InputInterfaceData.AI.accPedSens2  IndexOptions=Index vector (dialog)  Indices=1  OutputSizes=1
  Data Store Read2 : DataStoreRead  DataStoreName=ManualOutputInterfaceData  DataStoreElements=ManualOutputInterfaceData.Param_Man.Man_F_AccPedalManualMode  IndexOptions=Index vector (dialog)  Indices=1  OutputSizes=1
  Data Store Read3 : DataStoreRead  DataStoreName=ManualOutputInterfaceData  DataStoreElements=ManualOutputInterfaceData.Param_Man.Man_AccPedRampSpd#ManualOutputInterfaceData.Param_Man.Man_AccPedalLimit#ManualOutputInterfaceData.Param_Man.Man_AccPedalPressed  IndexOptions=Index vector (dialog)  Indices=1  OutputSizes=1
  Data Store Write2 : DataStoreWrite  DataStoreName=InputFunctionsData  DataStoreElements=InputFunctionsData.accPedalPos  IndexOptions=Index vector (dialog)  Indices=1  OutputSizes=1
  Function Caller1 : FunctionCaller  FunctionPrototype=pctValue = PedalValues.calcPedalSensValue(voltValue,minValue,maxValue)  InputArgumentSpecifications=<Enter example>  OutputArgumentSpecifications=<Enter example>
  Function Caller2 : FunctionCaller  FunctionPrototype=[pedalVal,errorSts] = PedalValues.validatePedalSensValue(fstValue,secValue)  InputArgumentSpecifications=<Enter example>  OutputArgumentSpecifications=<Enter example>
  Function Caller5 : FunctionCaller  FunctionPrototype=pctValue = PedalValues.calcPedalSensValue(voltValue,minValue,maxValue)  InputArgumentSpecifications=<Enter example>  OutputArgumentSpecifications=<Enter example>
  Gain : Gain  Gain=0.01
  MATLAB Function : MATLAB Function  TreatAsAtomicUnit=on
  Multiport Switch : MultiPortSwitch  DataPortOrder=Zero-based contiguous  Inputs=2  zeroidx=on  SaturateOnIntegerOverflow=off  InputSameDT=off
  Terminator1 : Terminator
  calcPedalSensDirect : Subsystem  TreatAsAtomicUnit=on
  validatePedalSensValue : Subsystem  TreatAsAtomicUnit=on
  wires:
  Constant3/1 -> Function Caller5/2
  Function Caller5/1 -> Function Caller2/1
  Function Caller2/2 -> Terminator1/1
  Function Caller1/1 -> Function Caller2/2
  Constant1/1 -> Function Caller1/2
  Constant2/1 -> Function Caller5/3
  Constant/1 -> Function Caller1/3
  Data Store Read/1 -> Function Caller5/1
  Data Store Read1/1 -> Function Caller1/1
  Function Caller2/1 -> Multiport Switch/2
  Multiport Switch/1 -> Data Store Write2/1
  Data Store Read2/1 -> Multiport Switch/1, MATLAB Function/1(AccPedMode)
  MATLAB Function/1(Man_AccPedLvl) -> Multiport Switch/3
  Data Store Read3/2 -> MATLAB Function/3(AccPedLim)
  Data Store Read3/3 -> MATLAB Function/4(AccPedPress)
  Data Store Read3/1 -> Gain/1
  Gain/1 -> MATLAB Function/2(AccPedRamp)

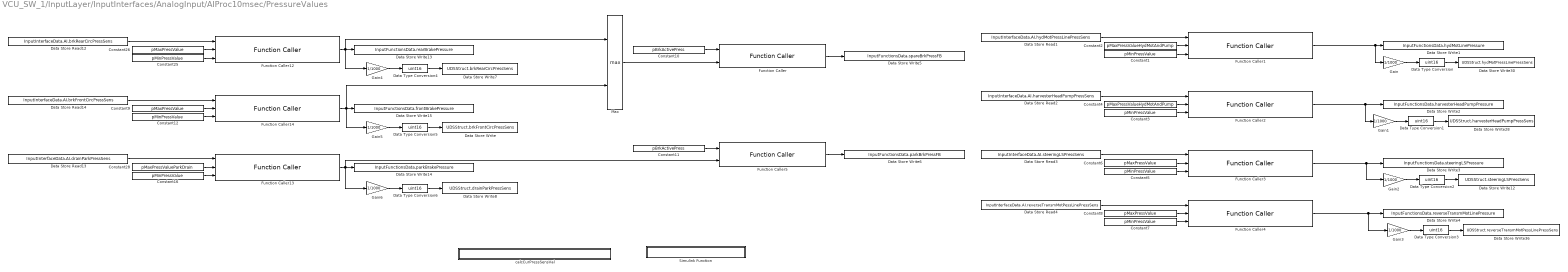
== system VCU_SW_1/InputLayer/InputInterfaces/AnalogInput/AIProc10msec/PressureValues ==
  Constant{1,3,5,7,12,16,25} (7 alike) : Constant  Value=pMinPressValue
  Constant10 : Constant  Value=pBrkActivePress
  Constant11 : Constant  Value=pBrkActivePress
  Constant2 : Constant  Value=pMaxPressValueHydMotAndPump
  Constant{6,8..9,26} (4 alike) : Constant  Value=pMaxPressValue
  Constant28 : Constant  Value=pMaxPressValueParkDrain
  Constant4 : Constant  Value=pMaxPressValueHydMotAndPump
  Data Store Read1 : DataStoreRead  DataStoreName=InputInterfaceData  DataStoreElements=InputInterfaceData.AI.hydMotPressLinePressSens  IndexOptions=Index vector (dialog)  Indices=1  OutputSizes=1
  Data Store Read12 : DataStoreRead  DataStoreName=InputInterfaceData  DataStoreElements=InputInterfaceData.AI.brkRearCircPressSens  IndexOptions=Index vector (dialog)  Indices=1  OutputSizes=1
  Data Store Read13 : DataStoreRead  DataStoreName=InputInterfaceData  DataStoreElements=InputInterfaceData.AI.drainParkPressSens  IndexOptions=Index vector (dialog)  Indices=1  OutputSizes=1
  Data Store Read14 : DataStoreRead  DataStoreName=InputInterfaceData  DataStoreElements=InputInterfaceData.AI.brkFrontCircPressSens  IndexOptions=Index vector (dialog)  Indices=1  OutputSizes=1
  Data Store Read2 : DataStoreRead  DataStoreName=InputInterfaceData  DataStoreElements=InputInterfaceData.AI.harvesterHeadPumpPressSens  IndexOptions=Index vector (dialog)  Indices=1  OutputSizes=1
  Data Store Read3 : DataStoreRead  DataStoreName=InputInterfaceData  DataStoreElements=InputInterfaceData.AI.steeringLSPressSens  IndexOptions=Index vector (dialog)  Indices=1  OutputSizes=1
  Data Store Read4 : DataStoreRead  DataStoreName=InputInterfaceData  DataStoreElements=InputInterfaceData.AI.reverseTransmMotPessLinePressSens  IndexOptions=Index vector (dialog)  Indices=1  OutputSizes=1
  Data Store Write : DataStoreWrite  DataStoreName=UDSStruct  DataStoreElements=UDSStruct.brkFrontCircPressSens  IndexOptions=Index vector (dialog)  Indices=1  OutputSizes=1
  Data Store Write1 : DataStoreWrite  DataStoreName=InputFunctionsData  DataStoreElements=InputFunctionsData.hydMotLinePressure  IndexOptions=Index vector (dialog)  Indices=1  OutputSizes=1
  Data Store Write12 : DataStoreWrite  DataStoreName=UDSStruct  DataStoreElements=UDSStruct.steeringLSPressSens  IndexOptions=Index vector (dialog)  Indices=1  OutputSizes=1
  Data Store Write13 : DataStoreWrite  DataStoreName=InputFunctionsData  DataStoreElements=InputFunctionsData.rearBrakePressure  IndexOptions=Index vector (dialog)  Indices=1  OutputSizes=1
  Data Store Write14 : DataStoreWrite  DataStoreName=InputFunctionsData  DataStoreElements=InputFunctionsData.parkBrakePressure  IndexOptions=Index vector (dialog)  Indices=1  OutputSizes=1
  Data Store Write15 : DataStoreWrite  DataStoreName=InputFunctionsData  DataStoreElements=InputFunctionsData.frontBrakePressure  IndexOptions=Index vector (dialog)  Indices=1  OutputSizes=1
  Data Store Write2 : DataStoreWrite  DataStoreName=InputFunctionsData  DataStoreElements=InputFunctionsData.harvesterHeadPumpPressure  IndexOptions=Index vector (dialog)  Indices=1  OutputSizes=1
  Data Store Write28 : DataStoreWrite  DataStoreName=UDSStruct  DataStoreElements=UDSStruct.harvesterHeadPumpPressSens  IndexOptions=Index vector (dialog)  Indices=1  OutputSizes=1
  Data Store Write3 : DataStoreWrite  DataStoreName=InputFunctionsData  DataStoreElements=InputFunctionsData.steeringLSPressure  IndexOptions=Index vector (dialog)  Indices=1  OutputSizes=1
  Data Store Write30 : DataStoreWrite  DataStoreName=UDSStruct  DataStoreElements=UDSStruct.hydMotPressLinePressSens  IndexOptions=Index vector (dialog)  Indices=1  OutputSizes=1
  Data Store Write36 : DataStoreWrite  DataStoreName=UDSStruct  DataStoreElements=UDSStruct.reverseTransmMotPessLinePressSens  IndexOptions=Index vector (dialog)  Indices=1  OutputSizes=1
  Data Store Write4 : DataStoreWrite  DataStoreName=InputFunctionsData  DataStoreElements=InputFunctionsData.reverseTransmMotLinePressure  IndexOptions=Index vector (dialog)  Indices=1  OutputSizes=1
  Data Store Write5 : DataStoreWrite  DataStoreName=InputFunctionsData  DataStoreElements=InputFunctionsData.spareBrkPressFB  IndexOptions=Index vector (dialog)  Indices=1  OutputSizes=1
  Data Store Write6 : DataStoreWrite  DataStoreName=InputFunctionsData  DataStoreElements=InputFunctionsData.parkBrkPressFB  IndexOptions=Index vector (dialog)  Indices=1  OutputSizes=1
  Data Store Write7 : DataStoreWrite  DataStoreName=UDSStruct  DataStoreElements=UDSStruct.brkRearCircPressSens  IndexOptions=Index vector (dialog)  Indices=1  OutputSizes=1
  Data Store Write8 : DataStoreWrite  DataStoreName=UDSStruct  DataStoreElements=UDSStruct.drainParkPressSens  IndexOptions=Index vector (dialog)  Indices=1  OutputSizes=1
  Data Type Conversion{,1..6} (7 alike) : DataTypeConversion  OutDataTypeStr=uint16  SaturateOnIntegerOverflow=off  RndMeth=Floor
  Function Caller : FunctionCaller  FunctionPrototype=stt = brkPressFBproc(pBrkActivePress,pressFB)  InputArgumentSpecifications=<Enter example>  OutputArgumentSpecifications=<Enter example>
  Function Caller{1..4,12..14} (7 alike) : FunctionCaller  FunctionPrototype=pressValue = PressureValues.calcCurPressSens(sensValue,pressMax,pressMin)  InputArgumentSpecifications=<Enter example>  OutputArgumentSpecifications=<Enter example>
  Function Caller5 : FunctionCaller  FunctionPrototype=stt = brkPressFBproc(pBrkActivePress,pressFB)  InputArgumentSpecifications=<Enter example>  OutputArgumentSpecifications=<Enter example>
  Gain{,1..6} (7 alike) : Gain  Gain=1/1000  OutDataTypeStr=Inherit: Same as input
  Max : MinMax  Function=max  Inputs=2
  Simulink Function : Subsystem  TreatAsAtomicUnit=on
  calcCurPressSensVal : Subsystem  TreatAsAtomicUnit=on
  wires:
  Constant25/1 -> Function Caller12/3
  Data Store Read12/1 -> Function Caller12/1
  Constant26/1 -> Function Caller12/2
  Constant16/1 -> Function Caller13/3
  Data Store Read13/1 -> Function Caller13/1
  Constant28/1 -> Function Caller13/2
  Constant9/1 -> Function Caller14/2
  Data Store Read14/1 -> Function Caller14/1
  Constant12/1 -> Function Caller14/3
  Data Store Read1/1 -> Function Caller1/1
  Constant2/1 -> Function Caller1/2
  Constant1/1 -> Function Caller1/3
  Data Store Read2/1 -> Function Caller2/1
  Constant4/1 -> Function Caller2/2
  Constant3/1 -> Function Caller2/3
  Data Store Read3/1 -> Function Caller3/1
  Constant6/1 -> Function Caller3/2
  Constant5/1 -> Function Caller3/3
  Data Store Read4/1 -> Function Caller4/1
  Constant8/1 -> Function Caller4/2
  Constant7/1 -> Function Caller4/3
  Max/1 -> Function Caller/2
  Constant10/1 -> Function Caller/1
  Function Caller/1 -> Data Store Write5/1
  Constant11/1 -> Function Caller5/1
  Function Caller5/1 -> Data Store Write6/1
  Gain/1 -> Data Type Conversion/1
  Function Caller1/1 -> Gain/1, Data Store Write1/1
  Data Type Conversion/1 -> Data Store Write30/1
  Gain1/1 -> Data Type Conversion1/1
  Function Caller2/1 -> Data Store Write2/1, Gain1/1
  Data Type Conversion1/1 -> Data Store Write28/1
  Gain2/1 -> Data Type Conversion2/1
  Function Caller3/1 -> Gain2/1, Data Store Write3/1
  Data Type Conversion2/1 -> Data Store Write12/1
  Gain3/1 -> Data Type Conversion3/1
  Function Caller4/1 -> Gain3/1, Data Store Write4/1
  Data Type Conversion3/1 -> Data Store Write36/1
  Gain4/1 -> Data Type Conversion4/1
  Function Caller12/1 -> Gain4/1, Max/1, Data Store Write13/1
  Data Type Conversion4/1 -> Data Store Write7/1
  Gain5/1 -> Data Type Conversion5/1
  Function Caller14/1 -> Gain5/1, Max/2, Data Store Write15/1
  Data Type Conversion5/1 -> Data Store Write/1
  Gain6/1 -> Data Type Conversion6/1
  Function Caller13/1 -> Gain6/1, Function Caller5/2, Data Store Write14/1
  Data Type Conversion6/1 -> Data Store Write8/1

== system VCU_SW_1/InputLayer/InputInterfaces/AnalogInput/AIProc10msec/PumpMotorDirections ==
  Data Store Read1 : DataStoreRead  DataStoreName=InputInterfaceData  DataStoreElements=InputInterfaceData.AI.transmPumpDirSens  IndexOptions=Index vector (dialog)  Indices=1  OutputSizes=1
  Data Store Read2 : DataStoreRead  DataStoreName=InputInterfaceData  DataStoreElements=InputInterfaceData.AI.transmMotDirSens  IndexOptions=Index vector (dialog)  Indices=1  OutputSizes=1
  Data Store Read3 : DataStoreRead  DataStoreName=InputInterfaceData  DataStoreElements=InputInterfaceData.PWD.transPumpSpdSensSig1  IndexOptions=Index vector (dialog)  Indices=1  OutputSizes=1
  Data Store Read4 : DataStoreRead  DataStoreName=InputInterfaceData  DataStoreElements=InputInterfaceData.PWD.transPumpSpdSensSig2  IndexOptions=Index vector (dialog)  Indices=1  OutputSizes=1
  Data Store Read8 : DataStoreRead  DataStoreName=InputInterfaceData  DataStoreElements=InputInterfaceData.PWD.transmHydMotSpdSensSig1  IndexOptions=Index vector (dialog)  Indices=1  OutputSizes=1
  Data Store Read9 : DataStoreRead  DataStoreName=InputInterfaceData  DataStoreElements=InputInterfaceData.PWD.transmHydMotSpdSensSig2  IndexOptions=Index vector (dialog)  Indices=1  OutputSizes=1
  Data Store Write1 : DataStoreWrite  DataStoreName=InputFunctionsData  DataStoreElements=InputFunctionsData.HMotorDir  IndexOptions=Index vector (dialog)  Indices=1  OutputSizes=1
  Data Store Write2 : DataStoreWrite  DataStoreName=InputFunctionsData  DataStoreElements=InputFunctionsData.HPumpDir  IndexOptions=Index vector (dialog)  Indices=1  OutputSizes=1
  Data Store Write37 : DataStoreWrite  DataStoreName=UDSStruct  DataStoreElements=UDSStruct.transmMotDirSens  IndexOptions=Index vector (dialog)  Indices=1  OutputSizes=1
  Data Store Write38 : DataStoreWrite  DataStoreName=UDSStruct  DataStoreElements=UDSStruct.transmPumpDirSens  IndexOptions=Index vector (dialog)  Indices=1  OutputSizes=1
  Data Type Conversion : DataTypeConversion  OutDataTypeStr=uint16  SaturateOnIntegerOverflow=off  RndMeth=Floor
  Data Type Conversion1 : DataTypeConversion  OutDataTypeStr=uint16  SaturateOnIntegerOverflow=off  RndMeth=Floor
  Function Caller1 : FunctionCaller  FunctionPrototype=RotDir = calcRotDirSens(sensValue,SpdSensSig1,SpdSensSig2)  InputArgumentSpecifications=<Enter example>  OutputArgumentSpecifications=<Enter example>
  Function Caller2 : FunctionCaller  FunctionPrototype=RotDir = calcRotDirSens(sensValue,SpdSensSig1,SpdSensSig2)  InputArgumentSpecifications=<Enter example>  OutputArgumentSpecifications=<Enter example>
  calcRotDirSens : Subsystem  TreatAsAtomicUnit=on
  wires:
  Function Caller2/1 -> Data Store Write1/1, Data Type Conversion1/1
  Function Caller1/1 -> Data Type Conversion/1, Data Store Write2/1
  Data Store Read1/1 -> Function Caller1/1
  Data Store Read3/1 -> Function Caller1/2
  Data Store Read4/1 -> Function Caller1/3
  Data Store Read2/1 -> Function Caller2/1
  Data Store Read8/1 -> Function Caller2/2
  Data Store Read9/1 -> Function Caller2/3
  Data Type Conversion/1 -> Data Store Write38/1
  Data Type Conversion1/1 -> Data Store Write37/1
